simulink model "Subsystem0"  (R2020b)
settings: Solver=VariableStepAuto  StartTime=0.0  StopTime=10.0  RelTol=1e-3
undefined symbols (not defined in the file): b, m
settings Model: Creator=amolg  LastModifiedBy=amolg
settings DataIOCC: SaveOutput=off  SaveTime=off

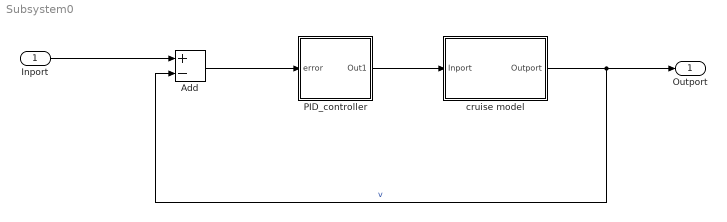
== system Subsystem0 ==
  Inport : Inport  OutDataTypeStr=double  PortDimensions=1  SampleTime=0
  Add : Sum  Inputs=+-
  PID_controller : Subsystem
  cruise model : Subsystem
  Outport : Outport  OutDataTypeStr=double  PortDimensions=1  SampleTime=0
  wires:
  cruise model/1(Outport) -> Add/2, Outport/1  "v"
  Inport/1 -> Add/1
  PID_controller/1(Out1) -> cruise model/1(Inport)
  Add/1 -> PID_controller/1(error)

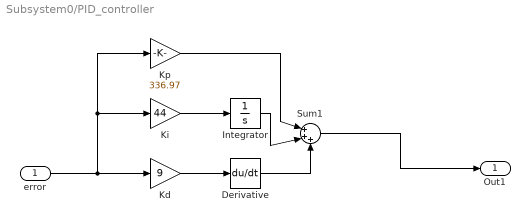
== system Subsystem0/PID_controller ==
  error : Inport  OutDataTypeStr=double  PortDimensions=1  SampleTime=0
  Derivative : Derivative
  Integrator : Integrator
  Kd : Gain  Gain=9
  Ki : Gain  Gain=44
  Kp : Gain  Gain=336.97
  Sum1 : Sum  Inputs=|+++
  Out1 : Outport  OutDataTypeStr=double  PortDimensions=1  SampleTime=0
  wires:
  Integrator/1 -> Sum1/2
  Kd/1 -> Derivative/1
  Ki/1 -> Integrator/1
  Kp/1 -> Sum1/1
  Derivative/1 -> Sum1/3
  Sum1/1 -> Out1/1
  error/1 -> Kp/1, Ki/1, Kd/1

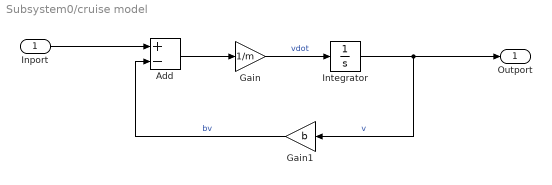
== system Subsystem0/cruise model ==
  Inport : Inport
  Add : Sum  Inputs=+-
  Gain : Gain  Gain=1/m
  Gain1 : Gain  Gain=b
  Integrator : Integrator
  Outport : Outport
  wires:
  Gain1/1 -> Add/2  "bv"
  Add/1 -> Gain/1
  Inport/1 -> Add/1
  Integrator/1 -> Gain1/1, Outport/1  "v"
  Gain/1 -> Integrator/1  "vdot"
